simulink model "dng_switching"  (Simulink 5.0)
settings: Solver=FixedStepDiscrete  StartTime=0.0  StopTime=inf  FixedStep=1e-1  RelTol=1e-3
libraries: dng_gmslib x1, dnglibv1 x1
settings Model: RequirementInfo=9  Creator=barnard  LastModifiedBy=howie  ExtModeTrigMode=oneshot  ExtModeArmWhenConnect=off  SaveTime=off  LimitDataPoints=off  BlockReductionOpt=off  BooleanDataType=off

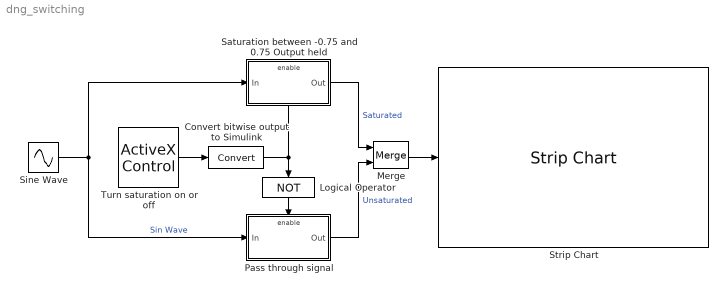
== system dng_switching ==
  Convert bitwise output to Simulink : DataTypeConversion  DataType=boolean  SaturateOnIntegerOverflow=on
  Logical Operator : Logic  Orientation=down  Operator=NOT
  Merge : Merge
  Pass through signal : Subsystem  TreatAsAtomicUnit=on
  Saturation between -0.75 and 0.75 Output held : Subsystem  TreatAsAtomicUnit=on
  Sine Wave : Sin  SampleTime=0
  Strip Chart : dng_gmslib/Strip Chart/Strip Chart  AncestorBlock=dnglibv1/ActiveX Control  progid=mwStrip.stripctrl.1  connect=input  init="hActx.TrackMin = -1.5; hActx.TrackDisplayMin = -1.5; hActx.TrackMax = 1.5; hActx.TrackDisplayMax = 1.5; hActx.XTicMode = 1; hActx.XSpan = 10/60/60/24; hActx.TimeSecondsFormat = '%M:%S'; hActx.TimeDateFormat = ''; hActx.TimeDaysFormat = ''; hActx.TimeHoursFormat = ''; hActx.TimeMinutesFormat = ''; hActx.TimeMonthsFormat = ''; hActx.TimeYearsFormat = ''; % Set x-axis to display time; set span = 10 sec (in fixed units=days); set display format = \"min:sec\" only"  inblock=on  border=on  dialOut=0
  Turn saturation on or off : dnglibv1/ActiveX Control  progid=mwtoggle.togglectrl.1  connect=output  output=Value  dialOutEvent=Click  init=hActx.configuration='Toggle Switch\Bitmap Toggles\OnOff Switch';  inblock=on  border=on  dialOut=0  updateParam=0
  wires:
  Turn saturation on or off/1 -> Convert bitwise output to Simulink/1
  Convert bitwise output to Simulink/1 -> Saturation between -0.75 and 0.75 Output held/Enable, Logical Operator/1
  Sine Wave/1 -> Saturation between -0.75 and 0.75 Output held/1(In), Pass through signal/1(In)  "Sin Wave"
  Saturation between -0.75 and 0.75 Output held/1(Out) -> Merge/1  "Saturated"
  Pass through signal/1(Out) -> Merge/2  "Unsaturated"
  Merge/1 -> Strip Chart/1
  Logical Operator/1 -> Pass through signal/Enable

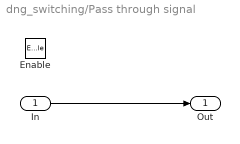
== system dng_switching/Pass through signal ==
  In : Inport
  Enable : EnablePort
  Out : Outport
  wires:
  In/1 -> Out/1

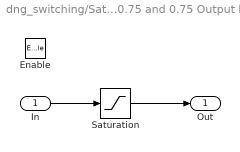
== system dng_switching/Saturation between -0.75 and 0.75 Output held ==
  In : Inport
  Enable : EnablePort
  Saturation : Saturate  UpperLimit=0.75  LowerLimit=-0.75
  Out : Outport
  wires:
  In/1 -> Saturation/1
  Saturation/1 -> Out/1
